simulink model "CompFilter"  (R2012b)
settings: Solver=FixedStepDiscrete  StartTime=0.0  StopTime=50  RelTol=1e-3
undefined symbols (not defined in the file): bw, Fs, gcbh, N, rmidispblock
libraries: FilterLib x4
settings Model: RequirementInfo={'other' '..\..\..\requirements\ebd_srs.doc' '@Simulink_requirement_item_4' 'true' 'REQ001- Filter input signal via polyphase digital filter bank' 'Requirement' } %GIDa_bfa4a348_cd9f_4101_a776_3ea215f34dae  RecordCoverage=on  Creator=aanantha  LastModifiedBy=klindqvi
settings DataIOCC: SaveFormat=Structure  SignalLoggingSaveFormat=ModelDataLogs  SaveOutput=off  SaveTime=off  SignalLoggingName=logsOut
settings OptimizationCC: InlineParams=on  OptimizeModelRefInitCode=on  LifeSpan=1
settings DebuggingCC: ReadBeforeWriteMsg=DisableAll  WriteAfterWriteMsg=DisableAll  WriteAfterReadMsg=DisableAll  SolverPrmCheckMsg=none  InheritedTsInSrcMsg=none  ParameterPrecisionLossMsg=none  FcnCallInpInsideContextMsg=EnableAllAsWarning
settings HardwareCC: ProdLargestAtomicInteger=Long  ProdLargestAtomicFloat=Double  ProdEndianess=LittleEndian  ProdHWDeviceType=ARM Compatible->ARM Cortex
settings RTWCC: SystemTargetFile=ert.tlc  TemplateMakefile=ert_default_tmf  Description=Embedded Coder  GenerateReport=on  RTWVerbose=off  ProcessScript=ert_make_rtw_hook  IncludeHyperlinkInReport=on  LaunchReport=on  PortableWordSizes=on  CodeProfilingSaveOptions=AllData  GenerateTraceInfo=on  GenerateTraceReportSl=on  GenerateTraceReportSf=on  GenerateTraceReportEml=on  GenerateCodeMetricsReport=on
settings CodeAppCC: IgnoreCustomStorageClasses=off
settings ERTTargetCC: CodeReplacementLibrary=GCC ARM Cortex-A8  MultiwordLength=2048  GenerateSampleERTMain=on  ERTCustomFileTemplate=example_file_process.tlc  ConvertIfToSwitch=off  SuppressUnreachableDefaultCases=off

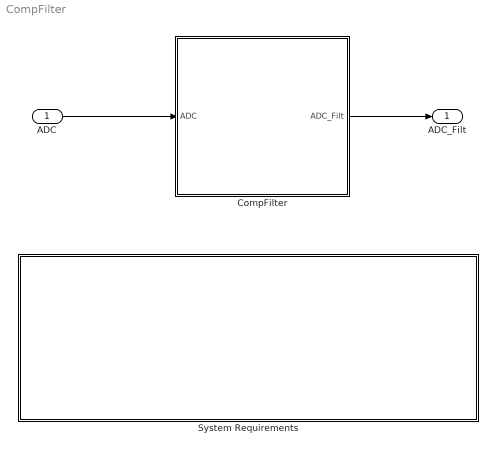
== system CompFilter ==
  ADC : Inport  OutDataTypeStr=single  PortDimensions=1  SampleTime=[0.001,0]
  CompFilter : Subsystem
  System Requirements : Subsystem  LoadFcn=rmidispblock('load',gcbh)  mask(System Requirements){id=SystemReq, title=System Requirements}
      mask prompts: title "Block Title"
      mask help: Lists the requirements for the current model.
      mask init:
      | id = 'SystemReq';
      | [w,h] = rmidispblock('display',gcbh);
      settings: CopyFcn=rmidispblock('create',gcbh)  DeleteFcn=rmidispblock('delete',gcbh)  ModelCloseFcn=rmidispblock('close',gcbh)  PreSaveFcn=rmidispblock('close',gcbh)  PostSaveFcn=rmidispblock('open',gcbh)  OpenFcn=rmidispblock('open',gcbh)  MoveFcn=rmidispblock('move',gcbh)
      mask Help: helpview(fullfile(docroot,'toolbox','slvnv','slvnv.map'),'systemrequirements')
      mask Display: text(w/2,h-4,rmidispblock('title',gcbh),'horizontalAlignment','center','verticalAlignment','top')
  ADC_Filt : Outport  OutDataTypeStr=single  PortDimensions=4  SampleTime=[0.08900000000000001,0]
  wires:
  ADC/1 -> CompFilter/1(ADC)
  CompFilter/1(ADC_Filt) -> ADC_Filt/1

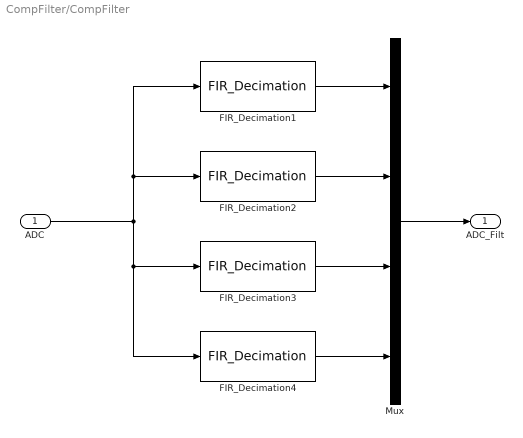
== system CompFilter/CompFilter ==
  ADC : Inport
  FIR_Decimation1 : FilterLib/FIR_Decimation  coefficients=fir1(N, (bw/(Fs/2))*[1 2])
  FIR_Decimation2 : FilterLib/FIR_Decimation  coefficients=fir1(N, (bw/(Fs/2))*[2 3])
  FIR_Decimation3 : FilterLib/FIR_Decimation  coefficients=fir1(N, (bw/(Fs/2))*[3 4])
  FIR_Decimation4 : FilterLib/FIR_Decimation  coefficients=fir1(N, (bw/(Fs/2))*[4 5])
  Mux : Mux
  ADC_Filt : Outport
  wires:
  Mux/1 -> ADC_Filt/1
  FIR_Decimation1/1 -> Mux/1
  FIR_Decimation2/1 -> Mux/2
  FIR_Decimation3/1 -> Mux/3
  FIR_Decimation4/1 -> Mux/4
  ADC/1 -> FIR_Decimation2/1, FIR_Decimation1/1, FIR_Decimation4/1, FIR_Decimation3/1

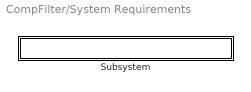
== system CompFilter/System Requirements ==
  Subsystem : Subsystem  mask{label=0, index=1}
      mask init:
      | label = rmidispblock('label',index);
      settings: OpenFcn=rmidispblock('openReq',gcbh);
      mask Display: text(0,0,label,'horizontalAlignment','left','verticalAlignment','bottom')

== system CompFilter/System Requirements/Subsystem ==
